simulink model "untitled"  (R2017a)
settings: Solver=VariableStepAuto  StartTime=0.0  StopTime=10.0  RelTol=1e-3
settings Model: Creator=mohammed  LastModifiedBy=mohammed

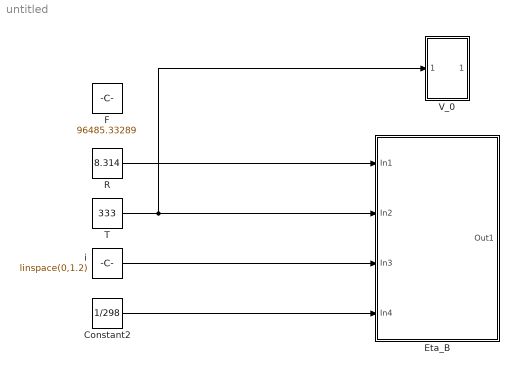
== system untitled ==
  Constant2 : Constant  Value=1/298
  Eta_B : Subsystem
  F : Constant  Value=96485.33289
  R : Constant  Value=8.314
  T : Constant  Value=333
  V_0 : Subsystem
  i : Constant  Value=linspace(0,1.2)
  wires:
  R/1 -> Eta_B/1(In1)
  i/1 -> Eta_B/3(In3)
  Constant2/1 -> Eta_B/4(In4)
  T/1 -> V_0/1(In1), Eta_B/2(In2)

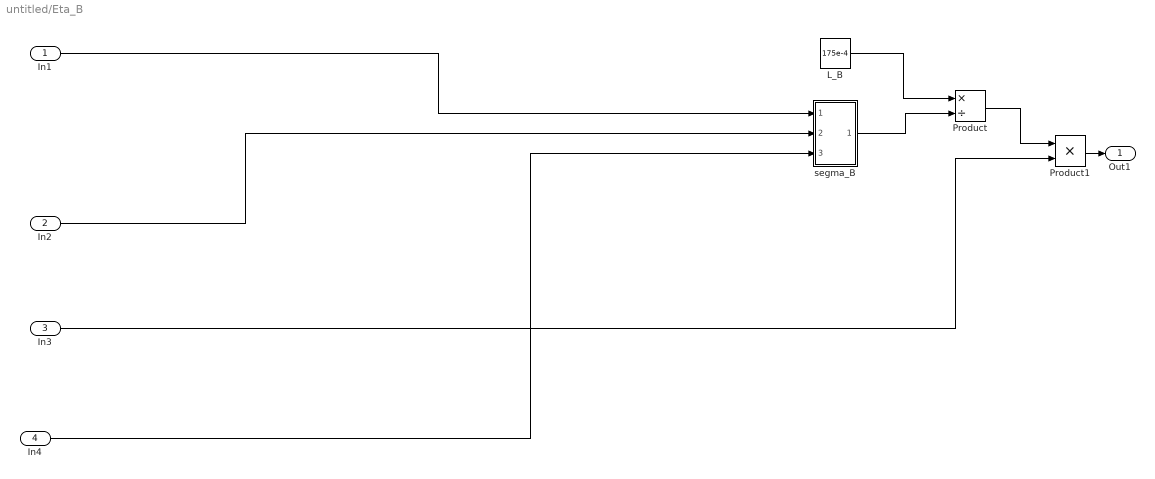
== system untitled/Eta_B ==
  In1 : Inport
  In2 : Inport  Port=2
  In3 : Inport  Port=3
  In4 : Inport  Port=4
  L_B : Constant  Value=175e-4
  Product : Product  Inputs=*/
  Product1 : Product
  segma_B : Subsystem
  Out1 : Outport
  wires:
  segma_B/1(Out1) -> Product/2
  L_B/1 -> Product/1
  Product1/1 -> Out1/1
  In3/1 -> Product1/2
  Product/1 -> Product1/1
  In2/1 -> segma_B/2(In2)
  In4/1 -> segma_B/3(In4)
  In1/1 -> segma_B/1(In1)

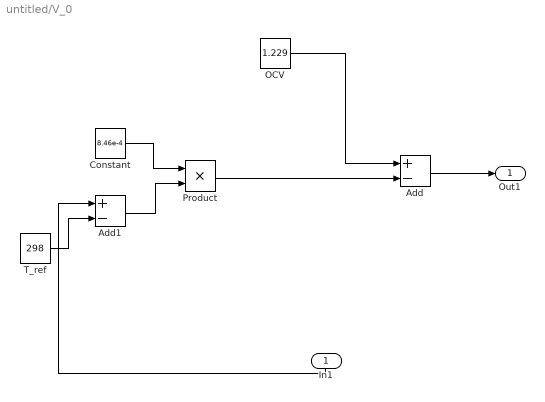
== system untitled/V_0 ==
  In1 : Inport
  Add : Sum  Inputs=+-
  Add1 : Sum  Inputs=+-
  Constant : Constant  Value=8.46e-4
  OCV : Constant  Value=1.229
  Product : Product
  T_ref : Constant  Value=298
  Out1 : Outport
  wires:
  OCV/1 -> Add/1
  Add/1 -> Out1/1
  Product/1 -> Add/2
  T_ref/1 -> Add1/2
  In1/1 -> Add1/1
  Constant/1 -> Product/1
  Add1/1 -> Product/2

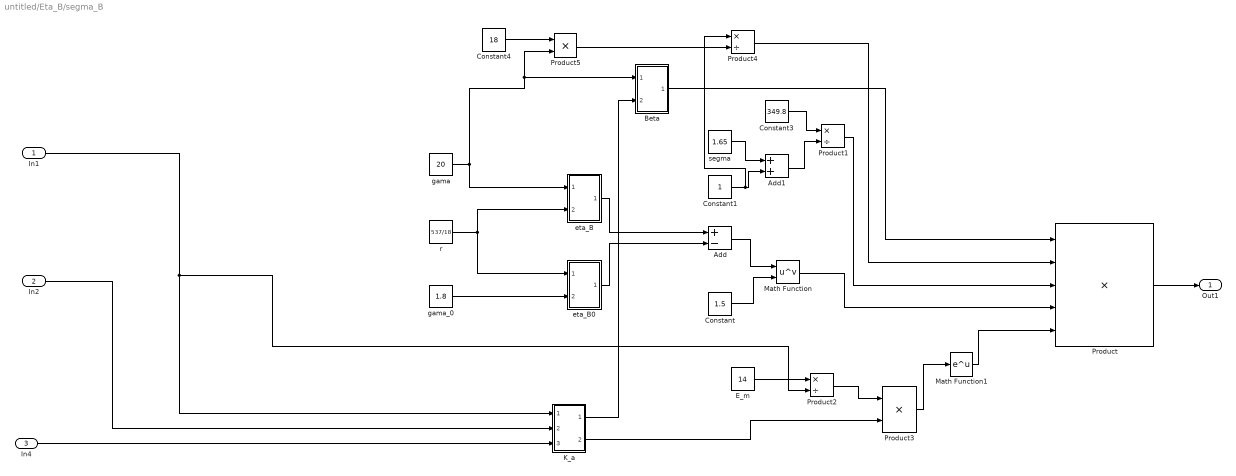
== system untitled/Eta_B/segma_B ==
  In1 : Inport
  In2 : Inport  Port=2
  In4 : Inport  Port=3
  Add : Sum  Inputs=+-
  Add1 : Sum
  Beta : Subsystem
  Constant : Constant  Value=1.5
  Constant1 : Constant
  Constant3 : Constant  Value=349.8
  Constant4 : Constant  Value=18
  E_m : Constant  Value=14
  K_a : Subsystem
  Math Function : Math  Operator=pow  SaturateOnIntegerOverflow=on
  Math Function1 : Math  SaturateOnIntegerOverflow=on
  Product : Product  Inputs=5
  Product1 : Product  Inputs=*/
  Product2 : Product  Inputs=*/
  Product3 : Product
  Product4 : Product  Inputs=*/
  Product5 : Product  Inputs=**
  eta_B : Subsystem
  eta_B0 : Subsystem
  gama : Constant  Value=20
  gama_0 : Constant  Value=1.8
  r : Constant  Value=537/18
  segma : Constant  Value=1.65
  Out1 : Outport
  wires:
  Constant1/1 -> Product4/1, Add1/2
  Math Function1/1 -> Product/5
  eta_B0/1(Out1) -> Add/2
  In4/1 -> K_a/3(In3)
  In1/1 -> Product2/2, K_a/1(In1)
  In2/1 -> K_a/2(In2)
  Product5/1 -> Product4/2
  K_a/1(Out1) -> Beta/2(In2)
  Constant3/1 -> Product1/1
  Math Function/1 -> Product/4
  E_m/1 -> Product2/1
  Constant/1 -> Math Function/2
  Add1/1 -> Product1/2
  segma/1 -> Add1/1
  Product1/1 -> Product/3
  gama_0/1 -> eta_B0/2(In2)
  Product3/1 -> Math Function1/1
  Add/1 -> Math Function/1
  Beta/1(Out1) -> Product/1
  Constant4/1 -> Product5/1
  Product4/1 -> Product/2
  gama/1 -> Product5/2, Beta/1(In1), eta_B/1(In1)
  r/1 -> eta_B0/1(In1), eta_B/2(In2)
  Product/1 -> Out1/1
  eta_B/1(Out1) -> Add/1
  K_a/2(Out2) -> Product3/2
  Product2/1 -> Product3/1

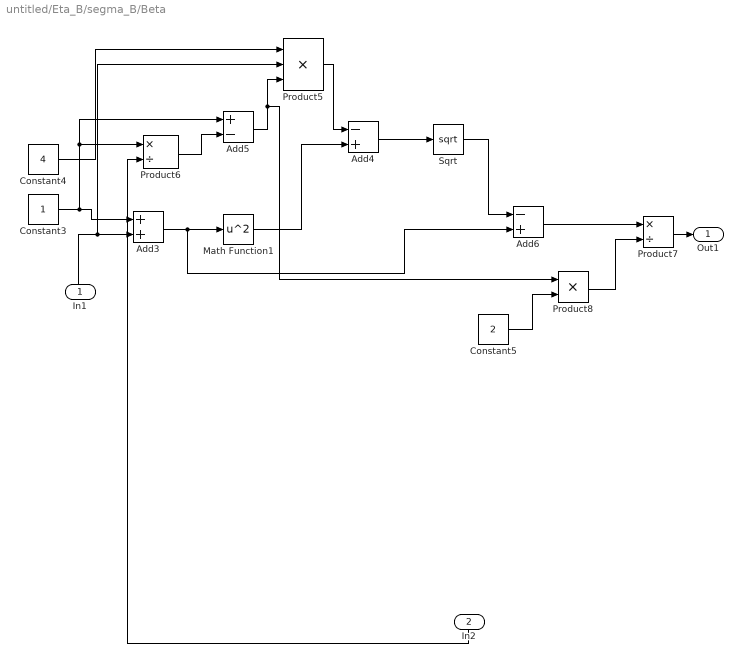
== system untitled/Eta_B/segma_B/Beta ==
  In1 : Inport
  In2 : Inport  Port=2
  Add3 : Sum
  Add4 : Sum  Inputs=-+
  Add5 : Sum  Inputs=+-
  Add6 : Sum  Inputs=-+
  Constant3 : Constant
  Constant4 : Constant  Value=4
  Constant5 : Constant  Value=2
  Math Function1 : Math  Operator=square  SaturateOnIntegerOverflow=on
  Product5 : Product  Inputs=***
  Product6 : Product  Inputs=*/
  Product7 : Product  Inputs=*/
  Product8 : Product  Inputs=**
  Sqrt : Sqrt  SaturateOnIntegerOverflow=on
  Out1 : Outport
  wires:
  Math Function1/1 -> Add4/2
  Constant3/1 -> Product6/1, Add5/1, Add3/1
  Add3/1 -> Add6/2, Math Function1/1
  Sqrt/1 -> Add6/1
  Constant4/1 -> Product5/1
  Constant5/1 -> Product8/2
  Add4/1 -> Sqrt/1
  Product6/1 -> Add5/2
  Product5/1 -> Add4/1
  Add6/1 -> Product7/1
  Product8/1 -> Product7/2
  Product7/1 -> Out1/1
  In1/1 -> Product5/2, Add3/2
  In2/1 -> Product6/2
  Add5/1 -> Product8/1, Product5/3

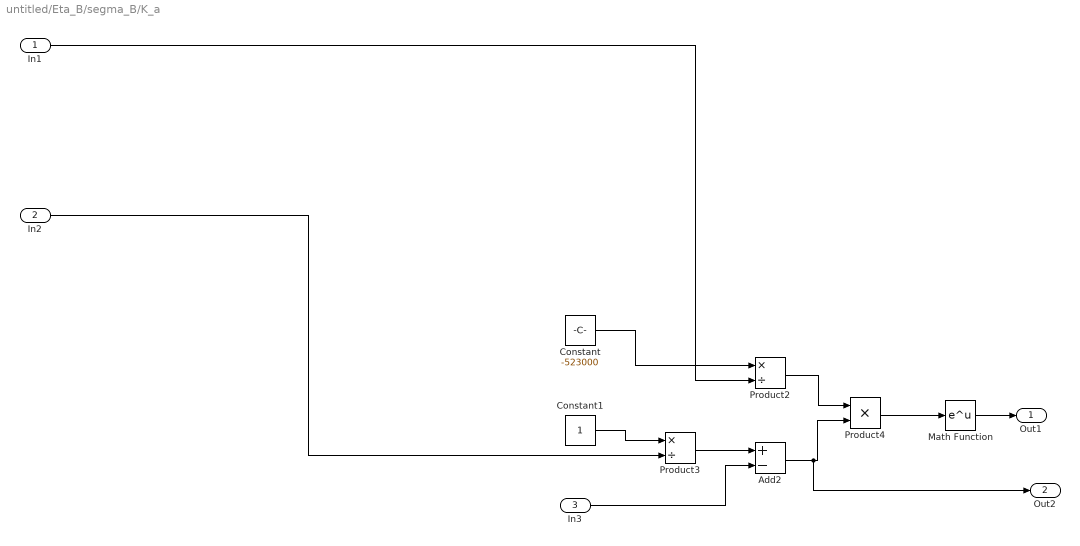
== system untitled/Eta_B/segma_B/K_a ==
  In1 : Inport
  In2 : Inport  Port=2
  In3 : Inport  Port=3
  Add2 : Sum  Inputs=+-
  Constant : Constant  Value=-523000
  Constant1 : Constant
  Math Function : Math  SaturateOnIntegerOverflow=on
  Product2 : Product  Inputs=*/
  Product3 : Product  Inputs=*/
  Product4 : Product
  Out1 : Outport
  Out2 : Outport  Port=2
  wires:
  Product4/1 -> Math Function/1
  Add2/1 -> Out2/1, Product4/2
  Math Function/1 -> Out1/1
  In3/1 -> Add2/2
  In2/1 -> Product3/2
  Product2/1 -> Product4/1
  Constant1/1 -> Product3/1
  Product3/1 -> Add2/1
  Constant/1 -> Product2/1
  In1/1 -> Product2/2

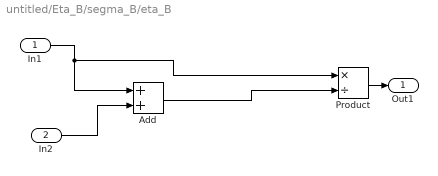
== system untitled/Eta_B/segma_B/eta_B ==
  In1 : Inport
  In2 : Inport  Port=2
  Add : Sum
  Product : Product  Inputs=*/
  Out1 : Outport
  wires:
  Product/1 -> Out1/1
  In2/1 -> Add/2
  In1/1 -> Product/1, Add/1
  Add/1 -> Product/2

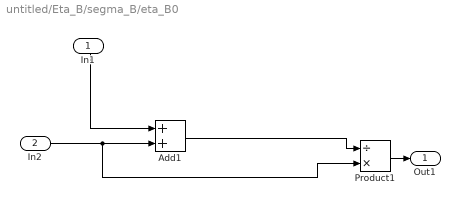
== system untitled/Eta_B/segma_B/eta_B0 ==
  In1 : Inport
  In2 : Inport  Port=2
  Add1 : Sum
  Product1 : Product  Inputs=/*
  Out1 : Outport
  wires:
  Add1/1 -> Product1/1
  Product1/1 -> Out1/1
  In1/1 -> Add1/1
  In2/1 -> Product1/2, Add1/2
